simulink model "untitled"  (R2018a)
settings: Solver=ode113  StartTime=0.0  StopTime=10.0  RelTol=1e-3
settings Model: Creator=sty  LastModifiedBy=sty

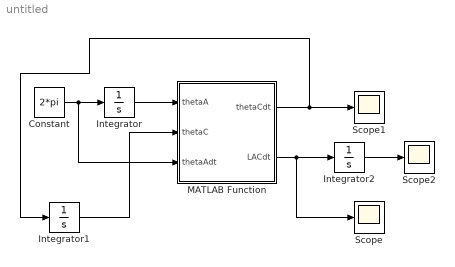
== system untitled ==
  Constant : Constant  Value=2*pi
  Integrator : Integrator
  Integrator1 : Integrator
  Integrator2 : Integrator  InitialCondition=5
  MATLAB Function : MATLAB Function  TreatAsAtomicUnit=on
  Scope : Scope
  Scope1 : Scope
  Scope2 : Scope
  wires:
  Constant/1 -> MATLAB Function/3(thetaAdt), Integrator/1
  MATLAB Function/1(thetaCdt) -> Integrator1/1, Scope1/1
  MATLAB Function/2(LACdt) -> Scope/1, Integrator2/1
  Integrator/1 -> MATLAB Function/1(thetaA)
  Integrator2/1 -> Scope2/1
  Integrator1/1 -> MATLAB Function/2(thetaC)

== matlab function untitled/MATLAB Function ==
  data: thetaA input; thetaCdt output; thetaC input; thetaAdt input; LACdt output
function [thetaCdt, LACdt] = fcn(thetaA, thetaC, thetaAdt)
LAB=1;
LBC=4;
thetaCdt = (LAB * thetaAdt * cos(thetaA)) / (LBC * cos(thetaC));
LACdt = -(LAB * thetaAdt * (cos(thetaA) * sin(thetaC) + cos(thetaC) *sin(thetaA))) / cos(thetaC);
end
